simulink library "LemmingToolbox"  (Simulink 7.0)
libraries: simulink x7, dspwin32 x4, viptextngfix x3, vrlib x1
settings Model: Creator=langmo  LastModifiedBy=langmo

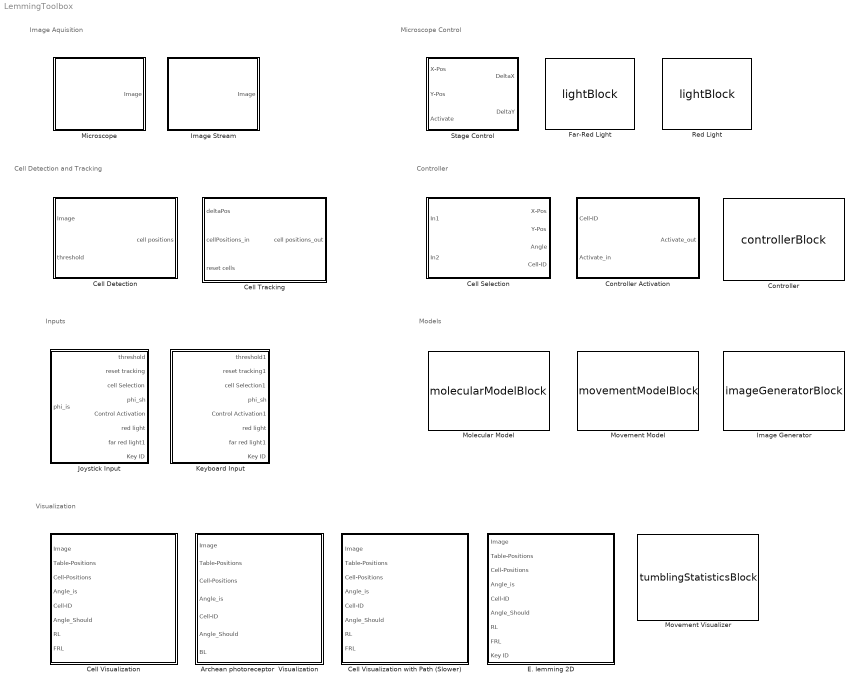
== system LemmingToolbox ==
  note: Image Aquisition
  note: Microscope Control
  note: Cell Detection and Tracking
  note: Controller
  note: Models
  note: Inputs
  note: Visualization
  Archean photoreceptor  Visualization : Subsystem  TreatAsAtomicUnit=on  SimViewingDevice=on  mask(Lemming Path Plotter){outputFilename=out.avi, imageDim=[1344,1024], binning=2, maxNumCells=1000, coneWidth=150, coneAngle=pi/4, pathLength=30, sampleTimes=[0.3, 0.1]}
      mask prompts: outputFilename "Output file name:"; imageDim "Original Image Dimensions:"; binning "Binning in Microscope:"; maxNumCells "Maximum Number of Cells:"; coneWidth "Cone Width:"; coneAngle "Cone Angle:"; pathLength "Path Length:"
      mask init:
      | [pic, map]=imread(fullfile(matlabroot,'/toolbox/LemmingToolbox/projector.jpg'));
      mask CallbackString:
      | fileName = get_param(gcb, 'outputFilename');
      | set_param([gcb, '/Save'], 'outputFilename', fileName);|||||||
      mask Display:
      | image(pic)
      | 
      | color('green');
      | port_label('input', 1, 'Image');
      | color('blue');
      | port_label('input', 2, 'Table-Positions');
      | port_label('input', 3, 'Cell-Positions');
      | port_label('input', 4, 'phi_is');
      | port_label('input', 5, 'Cell-ID');
      | color('red');
      | port_label('input', 6, 'phi_sh');
      | port_label('input', 7, 'BL');
  Cell Detection : Subsystem  mask(Cell Detection){imageDim=[1344,1024], binning=2, cellSizeLowerLimit=70, cellSizeUpperLimit=2000, maxNumCells=1000, resizeScale=0.5, sampleTimes=[0.3, 0.1]}
      mask prompts: imageDim "Original Image Dimensions:"; binning "Binning in Microscope:"; cellSizeLowerLimit "Lower Cell Size Limit:"; cellSizeUpperLimit "Upper Cell Size Limit"; maxNumCells "Maximum Number of Cells:"; resizeScale "Resize Factor:"
      mask help: Detects the cells in the image.
      mask init:
      | [data, map]=imread(fullfile(matlabroot,'/toolbox/LemmingToolbox/cellDetection.gif'));
      | pic=ind2rgb(data,map);
      mask Display:
      | image(pic)
      | color('blue');
      | port_label('output', 1, 'Cell-Positions');
      | color('green');
      | port_label('input', 1, 'Image');
      | color('red');
      | port_label('input', 2, 'threshold');
  Cell Selection : Subsystem  mask(Cell Tracking){numFrames=3, maxNumCells=1000, sampleTimes=[0.3, 0.1]}
      mask prompts: numFrames "Number of Frames to Determine Direction:"; maxNumCells "Maximum Number of Cells:"
      mask init:
      | [data, map]=imread(fullfile(matlabroot,'/toolbox/LemmingToolbox/cellTracking.gif'));
      | pic=ind2rgb(data,map);
      mask Display:
      | color('blue');
      | port_label('output', 1, 'X-Pos');
      | port_label('output', 2, 'Y-Pos');
      | port_label('output', 3, 'phi_is');
      | port_label('output', 4, 'Cell-ID');
      | port_label('input', 1, 'Cell-Positions');
      | color('red');
      | port_label('input', 2, 'Cell-Selection');
  Cell Tracking : Subsystem  mask(Cell Detection){maxDistance=0.05, maxNumCells=1000, tKeepLost=4, sampleTimes=[0.3, 0.1]}
      mask prompts: maxDistance "Maximal Travelling Distance:"; maxNumCells "Maximum Number of Cells:"; tKeepLost "Lost Cells Survival Time:"
      mask help: Detects the cells in the image.
      mask init:
      | [data, map]=imread(fullfile(matlabroot,'/toolbox/LemmingToolbox/cellTracking.gif'));
      | pic=ind2rgb(data,map);
      mask Display:
      | image(pic)
      | color('blue');
      | port_label('output', 1, 'Cell-Positions');
      | port_label('input', 1, 'Table-Position');
      | port_label('input', 2, 'Cell-Positions');
      | color('red');
      | port_label('input', 3, 'Reset Tracking');
  Cell Visualization : Subsystem  TreatAsAtomicUnit=on  SimViewingDevice=on  mask(Lemming Path Plotter){outputFilename=out.avi, imageDim=[1344,1024], binning=2, maxNumCells=1000, coneWidth=150, coneAngle=pi/4, pathLength=30, sampleTimes=[0.3, 0.1]}
      mask prompts: outputFilename "Output file name:"; imageDim "Original Image Dimensions:"; binning "Binning in Microscope:"; maxNumCells "Maximum Number of Cells:"; coneWidth "Cone Width:"; coneAngle "Cone Angle:"; pathLength "Path Length:"
      mask init:
      | [pic, map]=imread(fullfile(matlabroot,'/toolbox/LemmingToolbox/projector.jpg'));
      mask CallbackString:
      | fileName = get_param(gcb, 'outputFilename');
      | set_param([gcb, '/Save'], 'outputFilename', fileName);|||||||
      mask Display:
      | image(pic)
      | 
      | color('green');
      | port_label('input', 1, 'Image');
      | color('blue');
      | port_label('input', 2, 'Table-Positions');
      | port_label('input', 3, 'Cell-Positions');
      | port_label('input', 4, 'phi_is');
      | port_label('input', 5, 'Cell-ID');
      | color('red');
      | port_label('input', 6, 'phi_sh');
      | port_label('input', 7, 'RL');
      | port_label('input', 8, 'FRL');
  Cell Visualization with Path (Slower) : Subsystem  TreatAsAtomicUnit=on  SimViewingDevice=on  mask(Lemming Path Plotter){outputFilename=outWithPath.avi, imageDim=[1344,1024], binning=2, maxNumCells=1000, coneWidth=150, coneAngle=pi/4, pathLength=30, frameWidth=100, frameHeight=100, maxPathDimensions=[-2, -2, 12, 12], referenceX=[0, 0, 10, 10, 0], referenceY=[0, 10, 10, 0, 0], sampleTimes=[0.3, 0.1]}
      mask prompts: outputFilename "Output file name:"; imageDim "Original Image Dimensions:"; binning "Binning in Microscope:"; maxNumCells "Maximum Number of Cells:"; coneWidth "Cone Width:"; coneAngle "Cone Angle:"; pathLength "Path Length:"; frameWidth "Path frame width:"; frameHeight "Path frame heigth:"; maxPathDimensions "Maximal path dimensions:"; referenceX "Reference path corner x values:"; referenceY "Reference path corner y values:"
      mask init:
      | [pic, map]=imread(fullfile(matlabroot,'/toolbox/LemmingToolbox/projector.jpg'));
      mask CallbackString:
      | fileName = get_param(gcb, 'outputFilename');
      | set_param([gcb, '/Save'], 'outputFilename', fileName);||||||||||||
      mask Display:
      | image(pic)
      | 
      | color('green');
      | port_label('input', 1, 'Image');
      | color('blue');
      | port_label('input', 2, 'Table-Positions');
      | port_label('input', 3, 'Cell-Positions');
      | port_label('input', 4, 'phi_is');
      | port_label('input', 5, 'Cell-ID');
      | color('red');
      | port_label('input', 6, 'phi_sh');
      | port_label('input', 7, 'RL');
      | port_label('input', 8, 'FRL');
  Controller : M-S-Function  FunctionName=controllerBlock  Parameters=sampleTimes, controller  mask{sampleTimes=[0.3, 0.1], controller=@controllerMoritz}
      mask prompts: controller "Controller function:"
      mask Display:
      | color('blue');
      | port_label('input', 1, 'phi_is');
      | port_label('input', 2, 'phi_sh');
      | color('red');
      | port_label('input', 3, 'Control Active');
      | port_label('output', 1, 'RL');
      | port_label('output', 2, 'FRL');
  Controller Activation : Subsystem  mask{isOn=off}
      mask prompts: isOn "Is active at startup"
      mask Display:
      | color('blue');
      | port_label('input', 1, 'Cell-ID');
      | color('red');
      | port_label('input', 2, 'Activate Control');
      | port_label('output', 1, 'Control Active');
  E. lemming 2D : Subsystem  TreatAsAtomicUnit=on  SimViewingDevice=on  mask(Lemming Path Plotter){outputFilename=game.avi, imageDim=[1344,1024], binning=2, maxNumCells=1000, coneWidth=150, coneAngle=pi/4, pathLength=30, sampleTimes=[0.3, 0.1]}
      mask prompts: outputFilename "Output file name:"; imageDim "Original Image Dimensions:"; binning "Binning in Microscope:"; maxNumCells "Maximum Number of Cells:"; coneWidth "Cone Width:"; coneAngle "Cone Angle:"; pathLength "Path Length:"
      mask init:
      | [pic, map]=imread(fullfile(matlabroot,'/toolbox/LemmingToolbox/projector.jpg'));
      mask CallbackString:
      | fileName = get_param(gcb, 'outputFilename');
      | set_param([gcb, '/Save'], 'outputFilename', fileName);|||||||
      mask Display:
      | image(pic)
      | 
      | color('green');
      | port_label('input', 1, 'Image');
      | color('blue');
      | port_label('input', 2, 'Table-Positions');
      | port_label('input', 3, 'Cell-Positions');
      | port_label('input', 4, 'phi_is');
      | port_label('input', 5, 'Cell-ID');
      | color('red');
      | port_label('input', 6, 'phi_sh');
      | port_label('input', 7, 'RL');
      | port_label('input', 8, 'FRL');
      | port_label('input', 9, 'Key ID');
  Far-Red Light : M-S-Function  FunctionName=lightBlock  Parameters=false, sampleTimes, activated  mask{activated=off, sampleTimes=[0.3, 0.1]}
      mask Display:
      | image(imread(fullfile(matlabroot,'/toolbox/LemmingToolbox/redLight.jpg')))
      | color('white');
      | port_label('input', 1, 'On/Off');
  Image Generator : M-S-Function  FunctionName=imageGeneratorBlock  Parameters=sampleTime, binning,numCells  mask{binning=2, numCells=1, sampleTime=[0.3, 0.1]}
      mask prompts: numCells "Number of Cells:"; sampleTime "SampleTimes:"
      mask Display:
      | color('green');
      | port_label('output', 1, 'Image');
      | color('blue');
      | port_label('input', 1, 'X-Pos');
      | port_label('input', 2, 'Y-Pos');
      | port_label('input', 3, 'phi_is');
      | port_label('input', 4, 'Table-Position');
  Image Stream : Subsystem  mask(Microscope Connection){imageDir=matlabroot/toolbox/LemmingToolbox/dummyImages, binning=2, sampleTimes=[0.3,0.1]}
      mask prompts: imageDir "Image Directory:"
      mask Display:
      | image(imread(fullfile(matlabroot,'/toolbox/LemmingToolbox/microscope.jpg')))
      | color('green');
      | port_label('output', 1, 'Image');
  Joystick Input : Subsystem  SystemSampleTime=1  mask{minMaxThresh=[0.05, 0.2], sampleTimes=[0.1, 0]}
      mask prompts: minMaxThresh "Minimal and maximal Threshold"
      mask init:
      | joyImage=imread(fullfile(matlabroot,'/toolbox/LemmingToolbox/joystick.jpg'));
      mask Display:
      | image(joyImage);
      | 
      | color('blue');
      | port_label('input', 1, 'phi_is');
      | color('red');
      | port_label('output', 1, 'Threshold');
      | port_label('output', 2, 'Reset Tracking');
      | port_label('output', 3, 'Cell-Selection');
      | port_label('output', 4, 'phi_sh');
      | port_label('output', 5, 'Activate Control');
      | port_label('output', 6, 'Light 1');
      | port_label('output', 7, 'Light 2');
      | port_label('output', 8, 'Key ID');
  Keyboard Input : Subsystem  SystemSampleTime=1  mask(Keyboard Input){initThreshold=0.09, sampleTimes=[0.2, 0]}
      mask prompts: initThreshold "Initial Threshold"
      mask help:
      | Use right arrow (or 'w') and left arrow to rotate the reference direction clock and counter-clock wise.
      | Use arrow up or down to activate red or far-red light.
      | Use the keys '1', '2' ,'3' ,'4' ,'6' ,'7', '8' and '9' to set the reference direction directly (best usable with the numeric keypad).
      | Use '+' and '-' to adjust the threshold for cell detection.
      | Use return and backslash to activate or deactivate the controller.
      | Use 'q' and 'e' to swicht to the next cell left or right from the current one.
      | Use the key '5' or space for special actions.
      mask init:
      | keyImage=imread(fullfile(matlabroot,'/toolbox/LemmingToolbox/keyboard.jpg'));
      mask Display:
      | image(keyImage);
      | 
      | color('red');
      | port_label('output', 1, 'Threshold');
      | port_label('output', 2, 'Reset Tracking');
      | port_label('output', 3, 'Cell-Selection');
      | port_label('output', 4, 'phi_sh');
      | port_label('output', 5, 'Activate Control');
      | port_label('output', 6, 'Light 1');
      | port_label('output', 7, 'Light 2');
      | port_label('output', 8, 'Key ID');
  "Microscope " : Subsystem  mask(Microscope Connection){sampleTimes=[0.3,0.1]}
      mask Display:
      | image(imread(fullfile(matlabroot,'/toolbox/LemmingToolbox/microscope.jpg')))
      | color('green');
      | port_label('output', 1, 'Image');
  Molecular Model : M-S-Function  FunctionName=molecularModelBlock  Parameters=molecModel, controlledCheSpecies, cheSpeciesAttachedTo, asp, CheX, AnkerProt, Anker  mask{molecModel=Spiro, controlledCheSpecies=CheR, cheSpeciesAttachedTo=CheX-PhyB & PIF3-Anker, asp=1e-3, useOrgParameters=on, CheX=0.3, AnkerProt=10, Anker=13}
      mask prompts: molecModel "Molecular Model:"; controlledCheSpecies "Controlled Species:"; cheSpeciesAttachedTo "Light coupling:"; asp "Aspartate:"; useOrgParameters "Use original parameter set:"; CheX "Controlled species concentration"; AnkerProt "Anker protein concentration:"; Anker "Anker concentration:"
      mask StyleString: popup(Spiro|Mello),popup(CheR|CheB|CheY|CheZ),popup(CheX-PIF3 & PhyB-Anker|CheX-PhyB & PIF3-Anker),edit,checkbox,edit,edit,edit
      mask CallbackString:
      | if strcmpi(get_param(gcb, 'useOrgParameters'), 'off')
      |     return;
      | end
      | molecModel = get_param(gcb, 'molecModel');
      | controlledCheSpecies = get_param(gcb, 'controlledCheSpecies');
      | cheSpeciesAttachedToPhyB = strcmpi(get_param(gcb, 'cheSpeciesAttachedTo'), 'CheX-PhyB & PIF3-Anker');
      | p = molecularModel('parameters', molecModel, controlledCheSpecies, cheSpeciesAttachedToPhyB);
      | switch controlledCheSpecies
      |     case 'CheR'
      |         set_param(gcb, 'CheX', sprintf('%g', p.R_tot));
      |     case 'CheB'
      |         set_param(gcb, 'CheX', sprintf('%g', p.B_tot));
      |     case 'CheY'
      |         set_param(gcb, 'CheX', sprintf('%g', p.Y_tot));
      |     case 'CheZ'
      |         set_param(gcb, 'CheX', sprintf('%g', p.Z_tot));
      | end
      | set_param(gcb, 'AnkerProt', sprintf('%g', p.AnkerProt_tot));
      | set_param(gcb, 'Anker', sprintf('%g', p.Anker_tot));|if strcmpi(get_param(gcb, 'useOrgParameters'), 'off')
      |     return;
      | end
      | molecModel = get_param(gcb, 'molecModel');
      | controlledCheSpecies = get_param(gcb, 'controlledCheSpecies');
      | cheSpeciesAttachedToPhyB = strcmpi(get_param(gcb, 'cheSpeciesAttachedTo'), 'CheX-PhyB & PIF3-Anker');
      | p = molecularModel('parameters', molecModel, controlledCheSpecies, cheSpeciesAttachedToPhyB);
      | switch controlledCheSpecies
      |     case 'CheR'
      |         set_param(gcb, 'CheX', sprintf('%g', p.R_tot));
      |     case 'CheB'
      |         set_param(gcb, 'CheX', sprintf('%g', p.B_tot));
      |     case 'CheY'
      |         set_param(gcb, 'CheX', sprintf('%g', p.Y_tot));
      |     case 'CheZ'
      |         set_param(gcb, 'CheX', sprintf('%g', p.Z_tot));
      | end
      | set_param(gcb, 'AnkerProt', sprintf('%g', p.AnkerProt_tot));
      | set_param(gcb, 'Anker', sprintf('%g', p.Anker_tot));|||if strcmpi(get_param(gcb, 'useOrgParameters'), 'off')
      |     set_param(gcb,'MaskEnables',{'on', 'on','on', 'on', 'on','on','on','on'});
      |     return;
      | end
      | 
      | set_param(gcb,'MaskEnables',{'on', 'on','on', 'on', 'on','off','off','off'});
      | molecModel = get_param(gcb, 'molecModel');
      | controlledCheSpecies = get_param(gcb, 'controlledCheSpecies');
      | cheSpeciesAttachedToPhyB = strcmpi(get_param(gcb, 'cheSpeciesAttachedTo'), 'CheX-PhyB & PIF3-Anker');
      | p = molecularModel('parameters', molecModel, controlledCheSpecies, cheSpeciesAttachedToPhyB);
      | switch controlledCheSpecies
      |     case 'CheR'
      |         set_param(gcb, 'CheX', sprintf('%g', p.R_tot));
      |     case 'CheB'
      |         set_param(gcb, 'CheX', sprintf('%g', p.B_tot));
      |     case 'CheY'
      |         set_param(gcb, 'CheX', sprintf('%g', p.Y_tot));
      |     case 'CheZ'
      |         set_param(gcb, 'CheX', sprintf('%g', p.Z_tot));
      | end
      | set_param(gcb, 'AnkerProt', sprintf('%g', p.AnkerProt_tot));
      | set_param(gcb, 'Anker', sprintf('%g', p.Anker_tot));|||
      mask Display:
      | color('blue');
      | port_label('output', 1, 'CheYp');
      | port_label('output', 2, 'Bias');
      | color('red');
      | port_label('input', 1, 'RL');
      | port_label('input', 2, 'FRL');
  Movement Model : M-S-Function  FunctionName=movementModelBlock  Parameters=sampleTimes , imageDim(2), imageDim(1), binning, pixelSize, initialCondition  mask{imageDim=[1344,1024], binning=2, pixelSize=6.45 / 40, initialCondition=[0.5, 0.5, 0], sampleTimes=[0.03, 0]}
      mask prompts: imageDim "Original Image Dimensions:"; pixelSize "Pixel size (mu M):"; initialCondition "Initial Position [xpos, ypos, phi_is]:"
      mask Display:
      | color('blue');
      | port_label('input', 1, 'Bias');
      | port_label('output', 1, 'X-Pos');
      | port_label('output', 2, 'Y-Pos');
      | port_label('output', 3, 'phi_is');
      | port_label('output', 4, 'isRunning');
  Movement Visualizer : M-S-Function  FunctionName=tumblingStatisticsBlock  Parameters=sampleTimes, numPoints  mask{numPoints=1000, sampleTimes=[0.3, 0.1]}
      mask prompts: numPoints "Number of stored data points:"
      mask Display:
      | color('blue');
      | port_label('input', 1, 'X-Pos');
      | port_label('input', 2, 'Y-Pos');
      | port_label('input', 3, 'phi_is');
      | port_label('input', 4, 'isRunning');
      | color('red');
      | port_label('input', 5, 'phi_sh');
  Red Light : M-S-Function  FunctionName=lightBlock  Parameters=true, sampleTimes, activated  mask{activated=off, sampleTimes=[0.3, 0.1]}
      mask Display:
      | image(imread(fullfile(matlabroot,'/toolbox/LemmingToolbox/redLight.jpg')))
      | color('white');
      | port_label('input', 1, 'On/Off');
  Stage Control : Subsystem  mask{activate=on, controlMicroscope=off, cooldown=5, border=0.25, initialCondition=[0, 0], sampleTimes=[0.3, 0.1]}
      mask prompts: controlMicroscope "Control Microscope"; cooldown "Cooldown (s):"; initialCondition "Initial position [x, y]:"
      mask init:
      | [pic, map]=imread(fullfile(matlabroot,'/toolbox/LemmingToolbox/changePosition.jpg'));
      mask Display:
      | image(pic)
      | color('blue');
      | port_label('output', 1, 'Table X');
      | port_label('output', 2, 'Table Y');
      | port_label('input', 1, 'X-Pos');
      | port_label('input', 2, 'Y-Pos');
      | color('red');
      | port_label('input', 3, 'Activate');

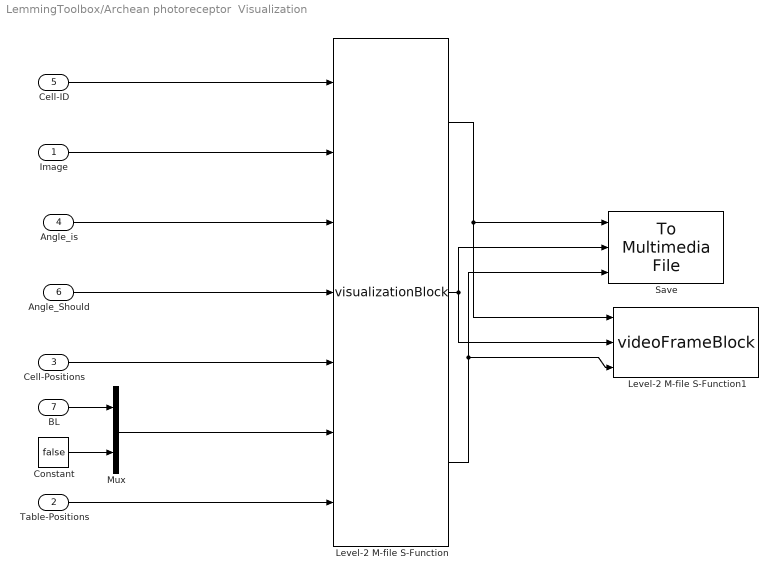
== system LemmingToolbox/Archean photoreceptor  Visualization ==
  Image : Inport  OutDataType=sfix(16)  OutScaling=2^0
  Table-Positions : Inport  Port=2  OutDataType=sfix(16)  OutScaling=2^0
  Cell-Positions : Inport  Port=3  OutDataType=sfix(16)  OutScaling=2^0
  Angle_is : Inport  Port=4  OutDataType=sfix(16)  OutScaling=2^0
  Cell-ID : Inport  Port=5  OutDataType=sfix(16)  OutScaling=2^0
  Angle_Should : Inport  Port=6  OutDataType=sfix(16)  OutScaling=2^0
  BL : Inport  Port=7  OutDataType=sfix(16)  OutScaling=2^0
  Constant : Constant  Value=false  OutDataType=sfix(16)  OutScaling=2^0
  Level-2 M-file S-Function : M-S-Function  FunctionName=visualizationBlock  Parameters=pathLength, coneWidth, coneAngle,3, sampleTimes, imageDim(1),imageDim(2), binning,maxNumCells
  Level-2 M-file S-Function1 : M-S-Function  FunctionName=videoFrameBlock  Parameters=sampleTimes
  Mux : Mux  Inputs=2
  Save : dspwin32/To Multimedia File  DialogController=dspDDGCreate  DialogControllerArgs=DataTag0  outputFilename=out.avi  streamSelection=Video only  videoCompressor=MJPEG Compressor  audioCompressor=None (uncompressed)  imagePorts=Separate color signals
  wires:
  BL/1 -> Mux/1
  Mux/1 -> Level-2 M-file S-Function/6
  Table-Positions/1 -> Level-2 M-file S-Function/7
  Cell-Positions/1 -> Level-2 M-file S-Function/5
  Angle_Should/1 -> Level-2 M-file S-Function/4
  Angle_is/1 -> Level-2 M-file S-Function/3
  Level-2 M-file S-Function/3 -> Level-2 M-file S-Function1/3, Save/3
  Level-2 M-file S-Function/2 -> Level-2 M-file S-Function1/2, Save/2
  Cell-ID/1 -> Level-2 M-file S-Function/1
  Image/1 -> Level-2 M-file S-Function/2
  Level-2 M-file S-Function/1 -> Level-2 M-file S-Function1/1, Save/1
  Constant/1 -> Mux/2

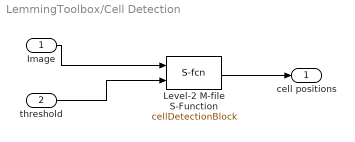
== system LemmingToolbox/Cell Detection ==
  Image : Inport  OutDataType=sfix(16)  OutScaling=2^0
  threshold : Inport  Port=2  OutDataType=sfix(16)  OutScaling=2^0
  Level-2 M-file S-Function : M-S-Function  FunctionName=cellDetectionBlock  Parameters=imageDim(1),imageDim(2),cellSizeLowerLimit,cellSizeUpperLimit,maxNumCells,resizeScale,binning, sampleTimes
  cell positions : Outport  OutDataType=sfix(16)  OutScaling=2^0
  wires:
  Image/1 -> Level-2 M-file S-Function/1
  Level-2 M-file S-Function/1 -> cell positions/1
  threshold/1 -> Level-2 M-file S-Function/2

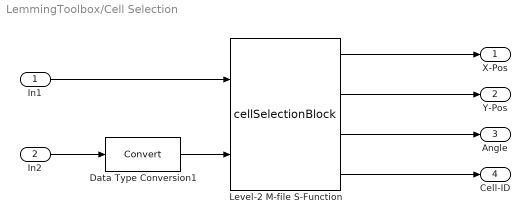
== system LemmingToolbox/Cell Selection ==
  In1 : Inport  OutDataType=sfix(16)  OutScaling=2^0
  In2 : Inport  Port=2  OutDataType=sfix(16)  OutScaling=2^0
  Data Type Conversion1 : DataTypeConversion  OutDataTypeMode=double  OutDataType=sfix(16)  OutScaling=2^0  SampleTime=sampleTimes
  Level-2 M-file S-Function : M-S-Function  FunctionName=cellSelectionBlock  Parameters=numFrames, sampleTimes, maxNumCells
  X-Pos : Outport  OutDataType=sfix(16)  OutScaling=2^0
  Y-Pos : Outport  Port=2  OutDataType=sfix(16)  OutScaling=2^0
  Angle : Outport  Port=3  OutDataType=sfix(16)  OutScaling=2^0
  Cell-ID : Outport  Port=4  OutDataType=sfix(16)  OutScaling=2^0
  wires:
  In1/1 -> Level-2 M-file S-Function/1
  In2/1 -> Data Type Conversion1/1
  Level-2 M-file S-Function/3 -> Angle/1
  Level-2 M-file S-Function/2 -> Y-Pos/1
  Level-2 M-file S-Function/1 -> X-Pos/1
  Data Type Conversion1/1 -> Level-2 M-file S-Function/2
  Level-2 M-file S-Function/4 -> Cell-ID/1

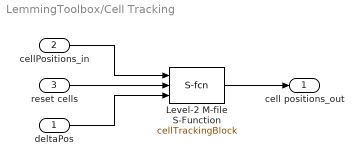
== system LemmingToolbox/Cell Tracking ==
  deltaPos : Inport  OutDataType=sfix(16)  OutScaling=2^0
  cellPositions_in : Inport  Port=2  OutDataType=sfix(16)  OutScaling=2^0
  reset cells : Inport  Port=3  OutDataType=sfix(16)  OutScaling=2^0
  Level-2 M-file S-Function : M-S-Function  FunctionName=cellTrackingBlock  Parameters=maxDistance, maxNumCells, tKeepLost, sampleTimes
  cell positions_out : Outport  OutDataType=sfix(16)  OutScaling=2^0
  wires:
  Level-2 M-file S-Function/1 -> cell positions_out/1
  cellPositions_in/1 -> Level-2 M-file S-Function/1
  reset cells/1 -> Level-2 M-file S-Function/2
  deltaPos/1 -> Level-2 M-file S-Function/3

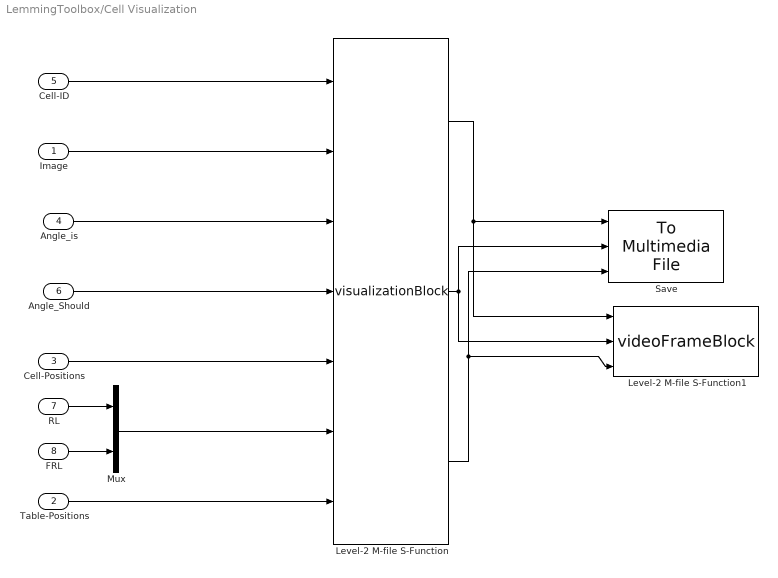
== system LemmingToolbox/Cell Visualization ==
  Image : Inport  OutDataType=sfix(16)  OutScaling=2^0
  Table-Positions : Inport  Port=2  OutDataType=sfix(16)  OutScaling=2^0
  Cell-Positions : Inport  Port=3  OutDataType=sfix(16)  OutScaling=2^0
  Angle_is : Inport  Port=4  OutDataType=sfix(16)  OutScaling=2^0
  Cell-ID : Inport  Port=5  OutDataType=sfix(16)  OutScaling=2^0
  Angle_Should : Inport  Port=6  OutDataType=sfix(16)  OutScaling=2^0
  RL : Inport  Port=7  OutDataType=sfix(16)  OutScaling=2^0
  FRL : Inport  Port=8  OutDataType=sfix(16)  OutScaling=2^0
  Level-2 M-file S-Function : M-S-Function  FunctionName=visualizationBlock  Parameters=pathLength, coneWidth, coneAngle,1, sampleTimes, imageDim(1),imageDim(2), binning,maxNumCells
  Level-2 M-file S-Function1 : M-S-Function  FunctionName=videoFrameBlock  Parameters=sampleTimes
  Mux : Mux  Inputs=2
  Save : dspwin32/To Multimedia File  DialogController=dspDDGCreate  DialogControllerArgs=DataTag1  outputFilename=out.avi  streamSelection=Video only  videoCompressor=MJPEG Compressor  audioCompressor=None (uncompressed)  imagePorts=Separate color signals
  wires:
  Level-2 M-file S-Function/1 -> Save/1, Level-2 M-file S-Function1/1
  Image/1 -> Level-2 M-file S-Function/2
  Cell-ID/1 -> Level-2 M-file S-Function/1
  Level-2 M-file S-Function/2 -> Save/2, Level-2 M-file S-Function1/2
  Level-2 M-file S-Function/3 -> Save/3, Level-2 M-file S-Function1/3
  Angle_is/1 -> Level-2 M-file S-Function/3
  Angle_Should/1 -> Level-2 M-file S-Function/4
  Cell-Positions/1 -> Level-2 M-file S-Function/5
  Table-Positions/1 -> Level-2 M-file S-Function/7
  Mux/1 -> Level-2 M-file S-Function/6
  RL/1 -> Mux/1
  FRL/1 -> Mux/2

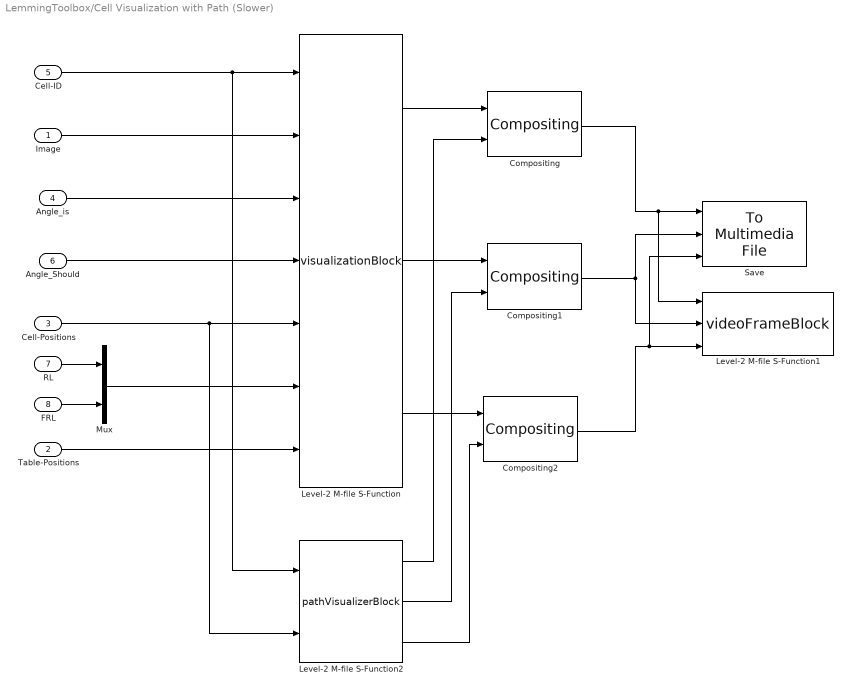
== system LemmingToolbox/Cell Visualization with Path (Slower) ==
  Image : Inport  OutDataType=sfix(16)  OutScaling=2^0
  Table-Positions : Inport  Port=2  OutDataType=sfix(16)  OutScaling=2^0
  Cell-Positions : Inport  Port=3  OutDataType=sfix(16)  OutScaling=2^0
  Angle_is : Inport  Port=4  OutDataType=sfix(16)  OutScaling=2^0
  Cell-ID : Inport  Port=5  OutDataType=sfix(16)  OutScaling=2^0
  Angle_Should : Inport  Port=6  OutDataType=sfix(16)  OutScaling=2^0
  RL : Inport  Port=7  OutDataType=sfix(16)  OutScaling=2^0
  FRL : Inport  Port=8  OutDataType=sfix(16)  OutScaling=2^0
  Compositing : viptextngfix/Compositing  DialogController=vipDDGCreate  DialogControllerArgs=DataTag2  operation=Blend  bFacSrc=Specify via dialog  mFacSrc=Specify via dialog  bFactor=0.3  mFactor=1  source=Specify via dialog  coordinates=[10, imageDim(1) / binning - frameWidth - 10]  prodOutputMode=Binary point scaling  prodOutputWordLength=32  prodOutputFracLength=10  roundingMode=Floor  overflowMode=off
  Compositing1 : viptextngfix/Compositing  DialogController=vipDDGCreate  DialogControllerArgs=DataTag3  operation=Blend  bFacSrc=Specify via dialog  mFacSrc=Specify via dialog  bFactor=0.3  mFactor=1  source=Specify via dialog  coordinates=[10, imageDim(1) / binning - frameWidth - 10]  prodOutputMode=Binary point scaling  prodOutputWordLength=32  prodOutputFracLength=10  roundingMode=Floor  overflowMode=off
  Compositing2 : viptextngfix/Compositing  DialogController=vipDDGCreate  DialogControllerArgs=DataTag4  operation=Blend  bFacSrc=Specify via dialog  mFacSrc=Specify via dialog  bFactor=0.3  mFactor=1  source=Specify via dialog  coordinates=[10, imageDim(1) / binning - frameWidth - 10]  prodOutputMode=Binary point scaling  prodOutputWordLength=32  prodOutputFracLength=10  roundingMode=Floor  overflowMode=off
  Level-2 M-file S-Function : M-S-Function  FunctionName=visualizationBlock  Parameters=pathLength, coneWidth, coneAngle,1, sampleTimes, imageDim(1),imageDim(2), binning,maxNumCells
  Level-2 M-file S-Function1 : M-S-Function  FunctionName=videoFrameBlock  Parameters=sampleTimes
  Level-2 M-file S-Function2 : M-S-Function  FunctionName=pathVisualizerBlock  Parameters=sampleTimes, frameWidth, frameHeight, maxNumCells, maxPathDimensions, referenceX, referenceY
  Mux : Mux  Inputs=2
  Save : dspwin32/To Multimedia File  DialogController=dspDDGCreate  DialogControllerArgs=DataTag5  outputFilename=outWithPath.avi  streamSelection=Video only  videoCompressor=MJPEG Compressor  audioCompressor=None (uncompressed)  imagePorts=Separate color signals
  wires:
  FRL/1 -> Mux/2
  RL/1 -> Mux/1
  Mux/1 -> Level-2 M-file S-Function/6
  Table-Positions/1 -> Level-2 M-file S-Function/7
  Cell-Positions/1 -> Level-2 M-file S-Function/5, Level-2 M-file S-Function2/2
  Angle_Should/1 -> Level-2 M-file S-Function/4
  Angle_is/1 -> Level-2 M-file S-Function/3
  Cell-ID/1 -> Level-2 M-file S-Function/1, Level-2 M-file S-Function2/1
  Image/1 -> Level-2 M-file S-Function/2
  Level-2 M-file S-Function/1 -> Compositing/1
  Level-2 M-file S-Function/2 -> Compositing1/1
  Level-2 M-file S-Function/3 -> Compositing2/1
  Level-2 M-file S-Function2/1 -> Compositing/2
  Level-2 M-file S-Function2/2 -> Compositing1/2
  Level-2 M-file S-Function2/3 -> Compositing2/2
  Compositing/1 -> Save/1, Level-2 M-file S-Function1/1
  Compositing2/1 -> Level-2 M-file S-Function1/3, Save/3
  Compositing1/1 -> Save/2, Level-2 M-file S-Function1/2

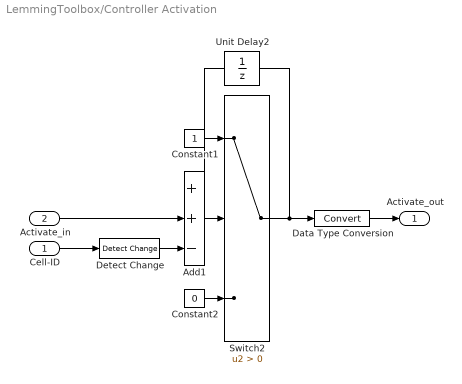
== system LemmingToolbox/Controller Activation ==
  Cell-ID : Inport  OutDataType=sfix(16)  OutScaling=2^0
  Activate_in : Inport  Port=2  OutDataType=sfix(16)  OutScaling=2^0
  Add1 : Sum  Inputs=++-  OutDataType=sfix(16)  OutScaling=2^-10
  Constant1 : Constant  OutDataType=sfix(16)  OutScaling=2^0
  Constant2 : Constant  Value=0  OutDataType=sfix(16)  OutScaling=2^0
  Data Type Conversion : DataTypeConversion  OutDataTypeMode=boolean  OutDataType=sfix(16)  OutScaling=2^0
  Detect Change : simulink/Logic and Bit Operations/Detect Change  SystemSampleTime=-1  vinit=0
  Switch2 : Switch  Criteria=u2 > Threshold  OutDataType=sfix(16)  OutScaling=2^0
  Unit Delay2 : UnitDelay  X0=isOn  SampleTime=-1
  Activate_out : Outport  OutDataType=sfix(16)  OutScaling=2^0
  wires:
  Switch2/1 -> Unit Delay2/1, Data Type Conversion/1
  Constant1/1 -> Switch2/1
  Constant2/1 -> Switch2/3
  Add1/1 -> Switch2/2
  Unit Delay2/1 -> Add1/1
  Activate_in/1 -> Add1/2
  Detect Change/1 -> Add1/3
  Cell-ID/1 -> Detect Change/1
  Data Type Conversion/1 -> Activate_out/1

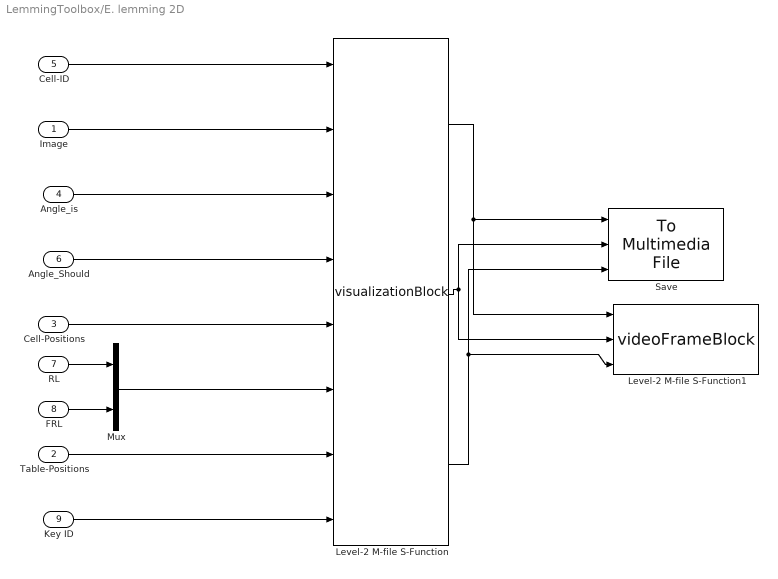
== system LemmingToolbox/E. lemming 2D ==
  Image : Inport  OutDataType=sfix(16)  OutScaling=2^0
  Table-Positions : Inport  Port=2  OutDataType=sfix(16)  OutScaling=2^0
  Cell-Positions : Inport  Port=3  OutDataType=sfix(16)  OutScaling=2^0
  Angle_is : Inport  Port=4  OutDataType=sfix(16)  OutScaling=2^0
  Cell-ID : Inport  Port=5  OutDataType=sfix(16)  OutScaling=2^0
  Angle_Should : Inport  Port=6  OutDataType=sfix(16)  OutScaling=2^0
  RL : Inport  Port=7  OutDataType=sfix(16)  OutScaling=2^0
  FRL : Inport  Port=8  OutDataType=sfix(16)  OutScaling=2^0
  Key ID : Inport  Port=9  OutDataType=sfix(16)  OutScaling=2^0
  Level-2 M-file S-Function : M-S-Function  FunctionName=visualizationBlock  Parameters=pathLength, coneWidth, coneAngle,2, sampleTimes, imageDim(1),imageDim(2), binning,maxNumCells
  Level-2 M-file S-Function1 : M-S-Function  FunctionName=videoFrameBlock  Parameters=sampleTimes
  Mux : Mux  Inputs=2
  Save : dspwin32/To Multimedia File  DialogController=dspDDGCreate  DialogControllerArgs=DataTag6  outputFilename=game.avi  streamSelection=Video only  videoCompressor=MJPEG Compressor  audioCompressor=None (uncompressed)  imagePorts=Separate color signals
  wires:
  FRL/1 -> Mux/2
  RL/1 -> Mux/1
  Mux/1 -> Level-2 M-file S-Function/6
  Table-Positions/1 -> Level-2 M-file S-Function/7
  Cell-Positions/1 -> Level-2 M-file S-Function/5
  Angle_Should/1 -> Level-2 M-file S-Function/4
  Angle_is/1 -> Level-2 M-file S-Function/3
  Level-2 M-file S-Function/3 -> Level-2 M-file S-Function1/3, Save/3
  Level-2 M-file S-Function/2 -> Level-2 M-file S-Function1/2, Save/2
  Cell-ID/1 -> Level-2 M-file S-Function/1
  Image/1 -> Level-2 M-file S-Function/2
  Level-2 M-file S-Function/1 -> Level-2 M-file S-Function1/1, Save/1
  Key ID/1 -> Level-2 M-file S-Function/8

== system LemmingToolbox/Image Stream ==
  Level-2 M-file S-Function : M-S-Function  FunctionName=imageStreamBlock  Parameters=binning,imageDir,sampleTimes
  Image : Outport  OutDataType=sfix(16)  OutScaling=2^0
  wires:
  Level-2 M-file S-Function/1 -> Image/1

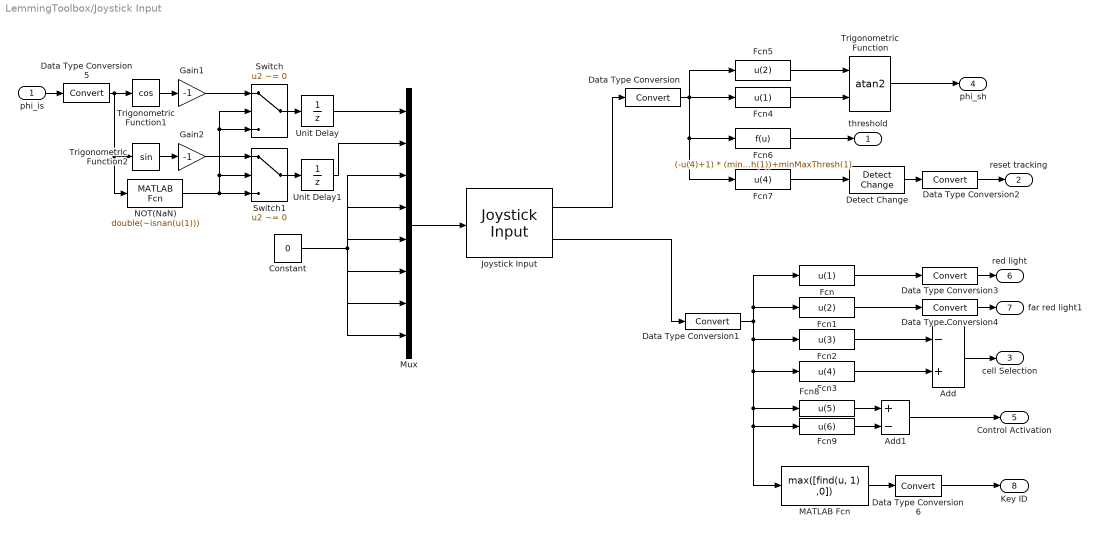
== system LemmingToolbox/Joystick Input ==
  phi_is : Inport  OutDataType=sfix(16)  OutScaling=2^0
  Add : Sum  Inputs=-+  OutDataType=sfix(16)  OutScaling=2^-10
  Add1 : Sum  Inputs=+-  OutDataType=sfix(16)  OutScaling=2^-10
  Constant : Constant  Value=0  OutDataType=sfix(16)  OutScaling=2^0
  Data Type Conversion : DataTypeConversion  OutDataTypeMode=double  OutDataType=sfix(16)  OutScaling=2^0  SampleTime=sampleTimes
  Data Type Conversion1 : DataTypeConversion  OutDataTypeMode=double  OutDataType=sfix(16)  OutScaling=2^0  SampleTime=sampleTimes
  Data Type Conversion2 : DataTypeConversion  OutDataTypeMode=boolean  OutDataType=sfix(16)  OutScaling=2^0
  Data Type Conversion3 : DataTypeConversion  OutDataTypeMode=boolean  OutDataType=sfix(16)  OutScaling=2^0
  Data Type Conversion4 : DataTypeConversion  OutDataTypeMode=boolean  OutDataType=sfix(16)  OutScaling=2^0
  Data Type Conversion5 : DataTypeConversion  OutDataTypeMode=double  OutDataType=sfix(16)  OutScaling=2^0  SampleTime=sampleTimes
  Data Type Conversion6 : DataTypeConversion  OutDataTypeMode=uint8  OutDataType=sfix(16)  OutScaling=2^0
  Detect Change : simulink/Logic and Bit Operations/Detect Change  SystemSampleTime=-1  vinit=0
  Fcn : Fcn  Expr=u(1)
  Fcn1 : Fcn  Expr=u(2)
  Fcn2 : Fcn  Expr=u(3)
  Fcn3 : Fcn  Expr=u(4)
  Fcn4 : Fcn  Expr=u(1)
  Fcn5 : Fcn  Expr=u(2)
  Fcn6 : Fcn  Expr=(-u(4)+1) * (minMaxThresh(2) - minMaxThresh(1))+minMaxThresh(1)
  Fcn7 : Fcn  Expr=u(4)
  Fcn8 : Fcn  Expr=u(5)
  Fcn9 : Fcn  Expr=u(6)
  Gain1 : Gain  Gain=-1  ParameterDataType=sfix(16)  ParameterScaling=2^0  OutDataType=sfix(16)  OutScaling=2^0
  Gain2 : Gain  Gain=-1  ParameterDataType=sfix(16)  ParameterScaling=2^0  OutDataType=sfix(16)  OutScaling=2^0
  Joystick Input : vrlib/Joystick Input  joyid=1  adjustports=off  forcefeed=on
  MATLAB Fcn : MATLABFcn  MATLABFcn=max([find(u, 1) ,0])
  Mux : Mux  Inputs=8
  NOT(NaN) : MATLABFcn  MATLABFcn=double(~isnan(u(1)))
  Switch : Switch  Criteria=u2 ~= 0  OutDataType=sfix(16)  OutScaling=2^0
  Switch1 : Switch  Criteria=u2 ~= 0  Threshold=0.5  OutDataType=sfix(16)  OutScaling=2^0
  Trigonometric Function : Trigonometry  Operator=atan2
  Trigonometric Function1 : Trigonometry  Operator=cos
  Trigonometric Function2 : Trigonometry
  Unit Delay : UnitDelay  SampleTime=-1
  Unit Delay1 : UnitDelay  SampleTime=-1
  threshold : Outport  OutDataType=sfix(16)  OutScaling=2^0
  reset tracking : Outport  Port=2  OutDataType=sfix(16)  OutScaling=2^0
  cell Selection : Outport  Port=3  OutDataType=sfix(16)  OutScaling=2^0
  phi_sh : Outport  Port=4  OutDataType=sfix(16)  OutScaling=2^0
  Control Activation : Outport  Port=5  OutDataType=sfix(16)  OutScaling=2^0
  red light : Outport  Port=6  OutDataType=sfix(16)  OutScaling=2^0
  far red light1 : Outport  Port=7  OutDataType=sfix(16)  OutScaling=2^0
  Key ID : Outport  Port=8  OutDataType=sfix(16)  OutScaling=2^0
  wires:
  Trigonometric Function/1 -> phi_sh/1
  Fcn6/1 -> threshold/1
  Add/1 -> cell Selection/1
  Fcn1/1 -> Data Type Conversion4/1
  Fcn/1 -> Data Type Conversion3/1
  Mux/1 -> Joystick Input/1
  Trigonometric Function1/1 -> Gain1/1
  Fcn2/1 -> Add/1
  Fcn3/1 -> Add/2
  Joystick Input/2 -> Data Type Conversion1/1
  Data Type Conversion1/1 -> Fcn2/1, Fcn3/1, Fcn8/1, Fcn9/1, MATLAB Fcn/1, Fcn1/1, Fcn/1
  Fcn4/1 -> Trigonometric Function/2
  Fcn5/1 -> Trigonometric Function/1
  Joystick Input/1 -> Data Type Conversion/1
  Constant/1 -> Mux/3, Mux/4, Mux/5, Mux/6, Mux/7, Mux/8
  phi_is/1 -> Data Type Conversion5/1
  Detect Change/1 -> Data Type Conversion2/1
  Fcn7/1 -> Detect Change/1
  Data Type Conversion2/1 -> reset tracking/1
  Gain1/1 -> Switch/1
  NOT(NaN)/1 -> Switch1/3, Switch/2, Switch/3, Switch1/2
  Switch/1 -> Unit Delay/1
  Switch1/1 -> Unit Delay1/1
  Trigonometric Function2/1 -> Gain2/1
  Data Type Conversion/1 -> Fcn4/1, Fcn5/1, Fcn6/1, Fcn7/1
  Data Type Conversion3/1 -> red light/1
  Data Type Conversion4/1 -> far red light1/1
  Data Type Conversion5/1 -> Trigonometric Function1/1, Trigonometric Function2/1, NOT(NaN)/1
  Unit Delay/1 -> Mux/1
  Unit Delay1/1 -> Mux/2
  Fcn9/1 -> Add1/2
  Fcn8/1 -> Add1/1
  Add1/1 -> Control Activation/1
  Gain2/1 -> Switch1/1
  MATLAB Fcn/1 -> Data Type Conversion6/1
  Data Type Conversion6/1 -> Key ID/1

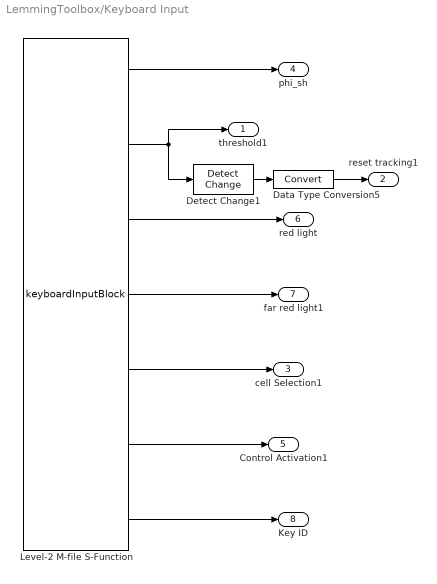
== system LemmingToolbox/Keyboard Input ==
  Data Type Conversion5 : DataTypeConversion  OutDataTypeMode=boolean  OutDataType=sfix(16)  OutScaling=2^0
  Detect Change1 : simulink/Logic and Bit Operations/Detect Change  SystemSampleTime=-1  vinit=0
  Level-2 M-file S-Function : M-S-Function  FunctionName=keyboardInputBlock  Parameters=sampleTimes, initThreshold
  threshold1 : Outport  OutDataType=sfix(16)  OutScaling=2^0
  reset tracking1 : Outport  Port=2  OutDataType=sfix(16)  OutScaling=2^0
  cell Selection1 : Outport  Port=3  OutDataType=sfix(16)  OutScaling=2^0
  phi_sh : Outport  Port=4  OutDataType=sfix(16)  OutScaling=2^0
  Control Activation1 : Outport  Port=5  OutDataType=sfix(16)  OutScaling=2^0
  red light : Outport  Port=6  OutDataType=sfix(16)  OutScaling=2^0
  far red light1 : Outport  Port=7  OutDataType=sfix(16)  OutScaling=2^0
  Key ID : Outport  Port=8  OutDataType=sfix(16)  OutScaling=2^0
  wires:
  Level-2 M-file S-Function/1 -> phi_sh/1
  Level-2 M-file S-Function/2 -> threshold1/1, Detect Change1/1
  Detect Change1/1 -> Data Type Conversion5/1
  Data Type Conversion5/1 -> reset tracking1/1
  Level-2 M-file S-Function/3 -> red light/1
  Level-2 M-file S-Function/4 -> far red light1/1
  Level-2 M-file S-Function/5 -> cell Selection1/1
  Level-2 M-file S-Function/6 -> Control Activation1/1
  Level-2 M-file S-Function/7 -> Key ID/1

== system LemmingToolbox/Microscope  ==
  Level-2 M-file S-Function : M-S-Function  FunctionName=microscopeBlock  Parameters=sampleTimes
  Image : Outport  OutDataType=sfix(16)  OutScaling=2^0
  wires:
  Level-2 M-file S-Function/1 -> Image/1

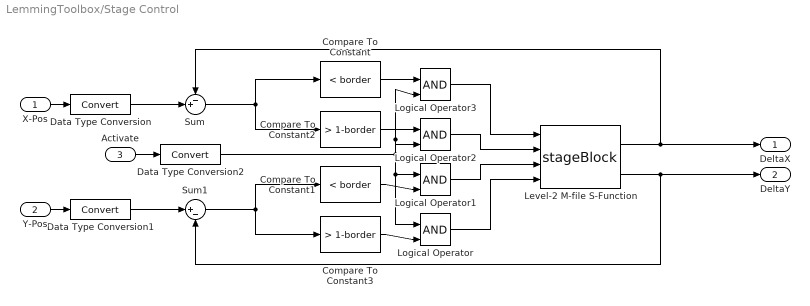
== system LemmingToolbox/Stage Control ==
  X-Pos : Inport  OutDataType=sfix(16)  OutScaling=2^0
  Y-Pos : Inport  Port=2  OutDataType=sfix(16)  OutScaling=2^0
  Activate : Inport  Port=3  OutDataType=sfix(16)  OutScaling=2^0
  Compare To Constant : simulink/Logic and Bit Operations/Compare To Constant  SystemSampleTime=-1  relop=<  const=border  LogicOutDataTypeMode=boolean  ZeroCross=off
  Compare To Constant1 : simulink/Logic and Bit Operations/Compare To Constant  SystemSampleTime=-1  relop=<  const=border  LogicOutDataTypeMode=boolean  ZeroCross=off
  Compare To Constant2 : simulink/Logic and Bit Operations/Compare To Constant  SystemSampleTime=-1  relop=>  const=1-border  LogicOutDataTypeMode=boolean  ZeroCross=off
  Compare To Constant3 : simulink/Logic and Bit Operations/Compare To Constant  SystemSampleTime=-1  relop=>  const=1-border  LogicOutDataTypeMode=boolean  ZeroCross=off
  Data Type Conversion : DataTypeConversion  OutDataTypeMode=double  OutDataType=sfix(16)  OutScaling=2^0  SampleTime=sampleTimes
  Data Type Conversion1 : DataTypeConversion  OutDataTypeMode=double  OutDataType=sfix(16)  OutScaling=2^0  SampleTime=sampleTimes
  Data Type Conversion2 : DataTypeConversion  OutDataTypeMode=boolean  OutDataType=sfix(16)  OutScaling=2^0  SampleTime=sampleTimes
  Level-2 M-file S-Function : M-S-Function  FunctionName=stageBlock  Parameters=cooldown, border, activate, controlMicroscope, initialCondition
  Logical Operator{,1..3} (4 alike) : Logic  IconShape=distinctive  AllPortsSameDT=off  OutDataTypeMode=boolean
  Sum : Sum  Inputs=-+|  OutDataType=sfix(16)  OutScaling=2^0
  Sum1 : Sum  Inputs=|+-  OutDataType=sfix(16)  OutScaling=2^0
  DeltaX : Outport  OutDataType=sfix(16)  OutScaling=2^0
  DeltaY : Outport  Port=2  OutDataType=sfix(16)  OutScaling=2^0
  wires:
  Level-2 M-file S-Function/1 -> Sum/1, DeltaX/1
  Level-2 M-file S-Function/2 -> Sum1/2, DeltaY/1
  X-Pos/1 -> Data Type Conversion/1
  Sum/1 -> Compare To Constant/1, Compare To Constant2/1
  Y-Pos/1 -> Data Type Conversion1/1
  Sum1/1 -> Compare To Constant1/1, Compare To Constant3/1
  Logical Operator/1 -> Level-2 M-file S-Function/4
  Logical Operator1/1 -> Level-2 M-file S-Function/3
  Logical Operator2/1 -> Level-2 M-file S-Function/2
  Logical Operator3/1 -> Level-2 M-file S-Function/1
  Compare To Constant/1 -> Logical Operator3/1
  Compare To Constant2/1 -> Logical Operator2/1
  Compare To Constant1/1 -> Logical Operator1/2
  Compare To Constant3/1 -> Logical Operator/2
  Activate/1 -> Data Type Conversion2/1
  Data Type Conversion/1 -> Sum/2
  Data Type Conversion1/1 -> Sum1/1
  Data Type Conversion2/1 -> Logical Operator1/1, Logical Operator/1, Logical Operator2/2, Logical Operator3/2
